simulink model "PSMG1"  (R2023b)
settings: Solver=ode23  StartTime=0.0  StopTime=1  FixedStep=0.0001  MaxStep=1e-4  RelTol=1e-3
undefined symbols (not defined in the file): J, Ke, Ld, Lq, p, Rs
settings Model: Creator=tudorn  LastModifiedBy=tudorn

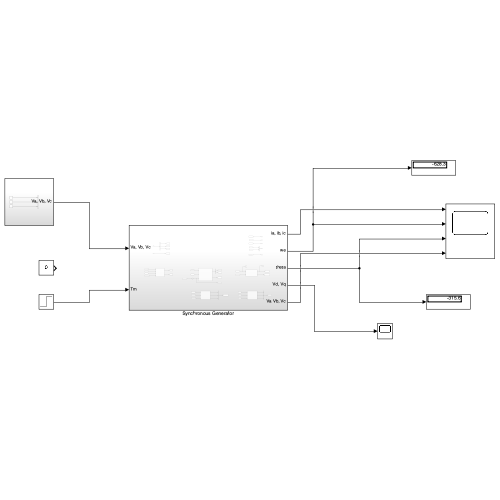
[thumbnail: Simulink's stored preview of the top-level diagram]
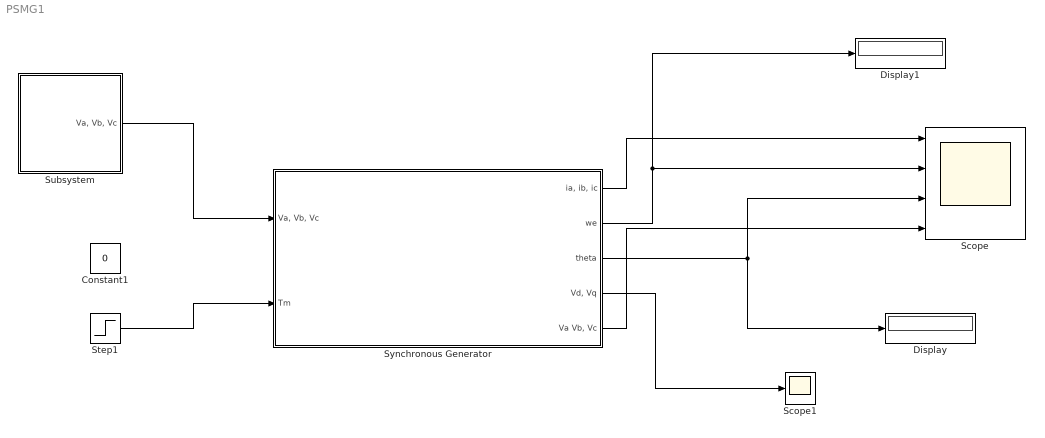
== system PSMG1 ==
  Constant1 : Constant  Value=0
  Display : Display
  Display1 : Display
  Scope : Scope  NumInputPorts=4
  Scope1 : Scope
  Step1 : Step  Time=0  After=3  SampleTime=0
  Subsystem : Subsystem
  Synchronous Generator : Subsystem
  wires:
  Subsystem/1("Va, Vb, Vc") -> Synchronous Generator/1("Va, Vb, Vc")
  Step1/1 -> Synchronous Generator/2(Tm)
  Synchronous Generator/1("ia, ib, ic") -> Scope/1
  Synchronous Generator/2(we) -> Display1/1, Scope/2
  Synchronous Generator/5("Va Vb, Vc") -> Scope/4
  Synchronous Generator/3(theta) -> Scope/3, Display/1
  Synchronous Generator/4("Vd, Vq") -> Scope1/1

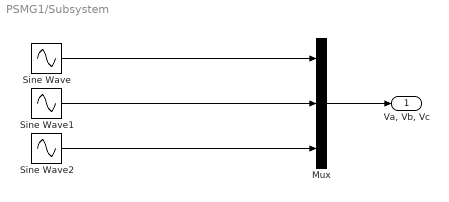
== system PSMG1/Subsystem ==
  Mux : Mux  Inputs=3
  Sine Wave : Sin  Amplitude=220  Frequency=2*pi*50  SampleTime=1e-5
  Sine Wave1 : Sin  Amplitude=220  Frequency=2*pi*50  Phase=2*pi/3  SampleTime=1e-5
  Sine Wave2 : Sin  Amplitude=220  Frequency=2*pi*50  Phase=-2*pi/3  SampleTime=1e-5
  "Va, Vb, Vc" : Outport
  wires:
  Mux/1 -> "Va, Vb, Vc"/1
  Sine Wave/1 -> Mux/1
  Sine Wave1/1 -> Mux/2
  Sine Wave2/1 -> Mux/3

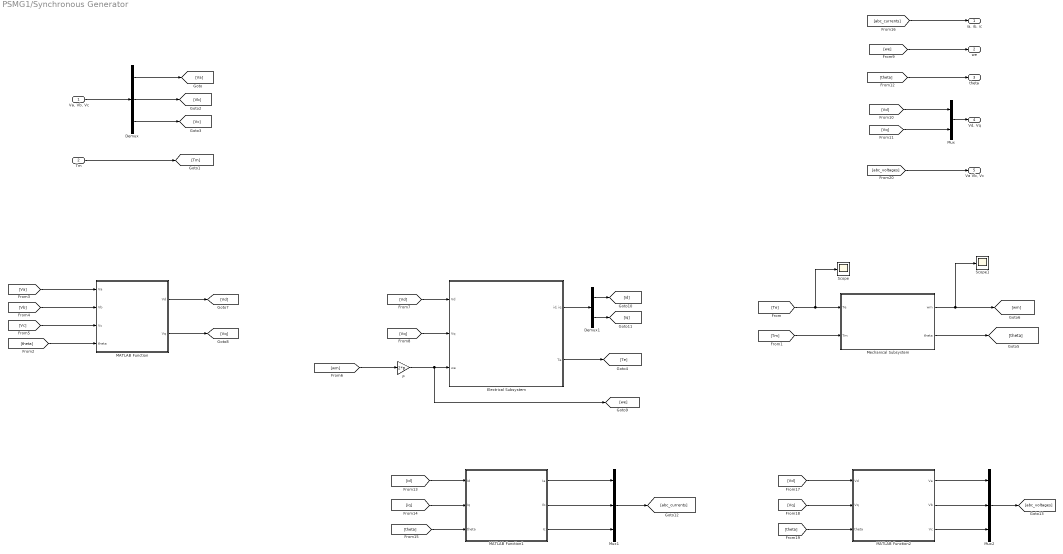
== system PSMG1/Synchronous Generator ==
  "Va, Vb, Vc" : Inport
  Tm : Inport  Port=2
  Demux : Demux  Outputs=3
  Demux1 : Demux  Outputs=2
  Electrical Subsystem : Subsystem
  MATLAB Function : MATLAB Function  TreatAsAtomicUnit=on
  MATLAB Function1 : MATLAB Function  TreatAsAtomicUnit=on
  MATLAB Function2 : MATLAB Function  TreatAsAtomicUnit=on
  Mechanical Subsystem : Subsystem
  Mux : Mux  Inputs=2
  Mux1 : Mux  Inputs=3
  Mux2 : Mux  Inputs=3
  P : Gain  Gain=2*p
  Scope : Scope
  Scope1 : Scope
  "ia, ib, ic" : Outport
  we : Outport  Port=2
  theta : Outport  Port=3
  "Vd, Vq" : Outport  Port=4
  "Va Vb, Vc" : Outport  Port=5
  wires:
  "Va, Vb, Vc"/1 -> Demux/1
  Tm/1 -> [Tm]
  Demux/1 -> [Va]
  Demux/2 -> [Vb]
  Demux/3 -> [Vc]
  Electrical Subsystem/2(Te) -> [Te]
  [Te] -> Scope/1, Mechanical Subsystem/1(Te)
  [Tm] -> Mechanical Subsystem/2(Tm)
  Mechanical Subsystem/2(theta) -> [theta]
  [theta] -> MATLAB Function/4(theta)
  [Vc] -> MATLAB Function/3(Vc)
  [Vb] -> MATLAB Function/2(Vb)
  [Va] -> MATLAB Function/1(Va)
  Mechanical Subsystem/1(wm) -> Scope1/1, [wm]
  [wm] -> P/1
  P/1 -> [we], Electrical Subsystem/3(we)
  [Vq] -> Electrical Subsystem/2(Vq)
  [Vd] -> Electrical Subsystem/1(Vd)
  MATLAB Function/1(Vd) -> [Vd]
  MATLAB Function/2(Vq) -> [Vq]
  [we] -> we/1
  Mux/1 -> "Vd, Vq"/1
  [Vd] -> Mux/1
  [Vq] -> Mux/2
  [theta] -> theta/1
  Electrical Subsystem/1("id, iq") -> Demux1/1
  Demux1/1 -> [id]
  Demux1/2 -> [iq]
  [iq] -> MATLAB Function1/2(Iq)
  [id] -> MATLAB Function1/1(Id)
  [theta] -> MATLAB Function1/3(theta)
  MATLAB Function1/1(Ia) -> Mux1/1
  MATLAB Function1/2(Ib) -> Mux1/2
  MATLAB Function1/3(Ic) -> Mux1/3
  Mux1/1 -> [abc_currents]
  [abc_currents] -> "ia, ib, ic"/1
  [Vd] -> MATLAB Function2/1(Vd)
  [Vq] -> MATLAB Function2/2(Vq)
  [theta] -> MATLAB Function2/3(theta)
  MATLAB Function2/1(Va) -> Mux2/1
  MATLAB Function2/2(Vb) -> Mux2/2
  MATLAB Function2/3(Vc) -> Mux2/3
  Mux2/1 -> [abc_voltages]
  [abc_voltages] -> "Va Vb, Vc"/1

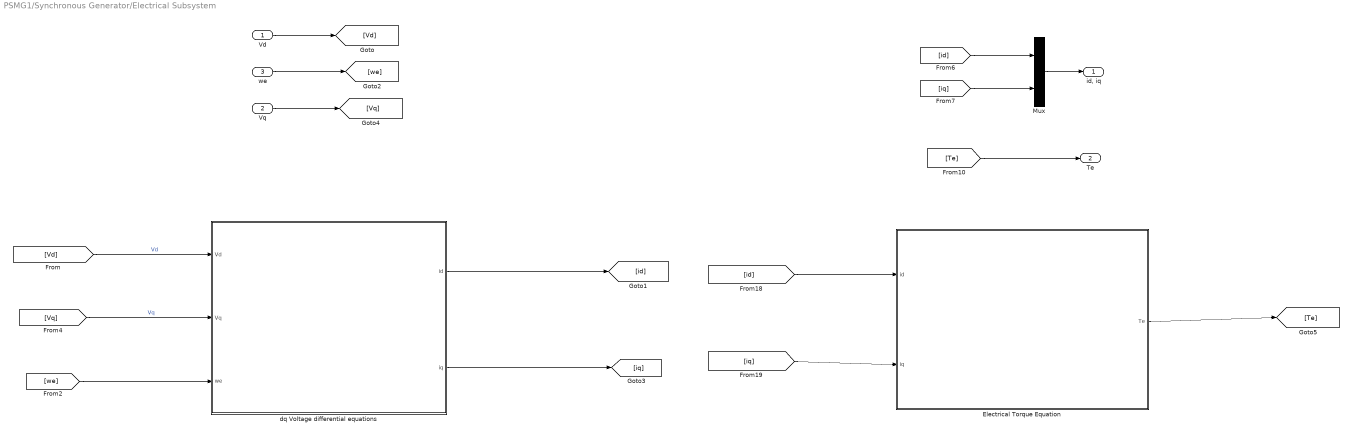
== system PSMG1/Synchronous Generator/Electrical Subsystem ==
  Vd : Inport
  Vq : Inport  Port=2
  we : Inport  Port=3
  Electrical Torque Equation : Subsystem
  Mux : Mux  Inputs=2
  dq Voltage differential equations : Subsystem
  "id, iq" : Outport
  Te : Outport  Port=2
  wires:
  Vd/1 -> [Vd]
  we/1 -> [we]
  Vq/1 -> [Vq]
  Mux/1 -> "id, iq"/1
  [id] -> Mux/1
  [iq] -> Mux/2
  [Te] -> Te/1
  [Vd] -> dq Voltage differential equations/1(Vd)  "Vd"
  [Vq] -> dq Voltage differential equations/2(Vq)  "Vq"
  dq Voltage differential equations/1(id) -> [id]
  dq Voltage differential equations/2(iq) -> [iq]
  [id] -> Electrical Torque Equation/1(id)
  [iq] -> Electrical Torque Equation/2(iq)
  Electrical Torque Equation/1(Te) -> [Te]
  [we] -> dq Voltage differential equations/3(we)

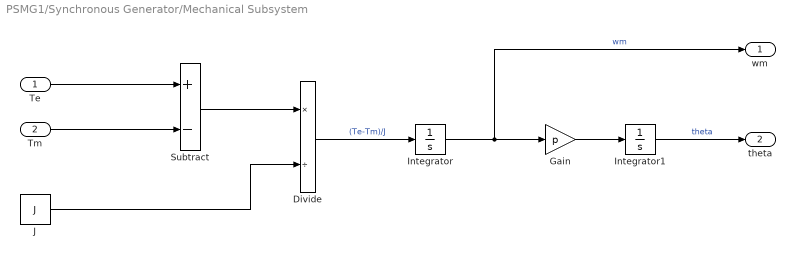
== system PSMG1/Synchronous Generator/Mechanical Subsystem ==
  Te : Inport
  Tm : Inport  Port=2
  Divide : Product  Inputs=*/
  Gain : Gain  Gain=p
  Integrator : Integrator
  Integrator1 : Integrator
  J : Constant  Value=J
  Subtract : Sum  Inputs=+-
  wm : Outport
  theta : Outport  Port=2
  wires:
  Tm/1 -> Subtract/2
  Te/1 -> Subtract/1
  Subtract/1 -> Divide/1
  J/1 -> Divide/2
  Divide/1 -> Integrator/1  "(Te-Tm)/J"
  Integrator/1 -> Gain/1, wm/1  "wm"
  Integrator1/1 -> theta/1  "theta"
  Gain/1 -> Integrator1/1

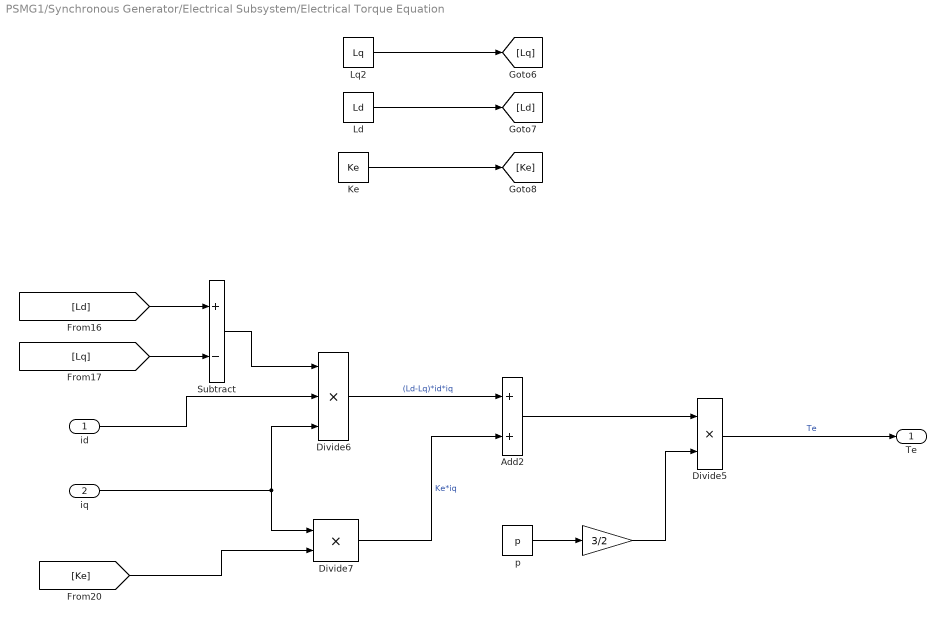
== system PSMG1/Synchronous Generator/Electrical Subsystem/Electrical Torque Equation ==
  id : Inport
  iq : Inport  Port=2
  " " : Gain  Gain=3/2
  Add2 : Sum
  Divide5 : Product  Inputs=**
  Divide6 : Product  Inputs=***
  Divide7 : Product  Inputs=**
  Ke : Constant  Value=Ke
  Ld : Constant  Value=Ld
  Lq2 : Constant  Value=Lq
  Subtract : Sum  Inputs=+-
  p : Constant  Value=p
  Te : Outport
  wires:
  id/1 -> Divide6/2
  [Ke] -> Divide7/2
  Divide5/1 -> Te/1  "Te"
  " "/1 -> Divide5/2
  iq/1 -> Divide7/1, Divide6/3
  [Ld] -> Subtract/1
  Subtract/1 -> Divide6/1
  p/1 -> " "/1
  Add2/1 -> Divide5/1
  Divide6/1 -> Add2/1  "(Ld-Lq)*id*iq"
  [Lq] -> Subtract/2
  Divide7/1 -> Add2/2  "Ke*iq"
  Ld/1 -> [Ld]
  Lq2/1 -> [Lq]
  Ke/1 -> [Ke]

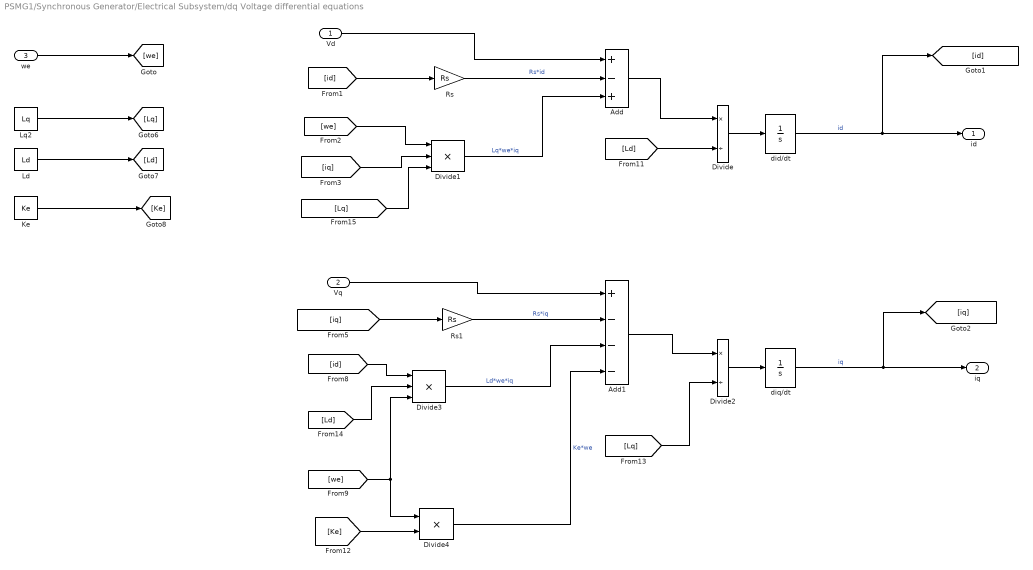
== system PSMG1/Synchronous Generator/Electrical Subsystem/dq Voltage differential equations ==
  Vd : Inport
  Vq : Inport  Port=2
  we : Inport  Port=3
  Add : Sum  Inputs=+-+
  Add1 : Sum  Inputs=+---
  Divide : Product  Inputs=*/
  Divide1 : Product  Inputs=***
  Divide2 : Product  Inputs=*/
  Divide3 : Product  Inputs=***
  Divide4 : Product  Inputs=**
  Ke : Constant  Value=Ke
  Ld : Constant  Value=Ld
  Lq2 : Constant  Value=Lq
  Rs : Gain  Gain=Rs
  Rs1 : Gain  Gain=Rs
  did/dt : Integrator
  diq/dt : Integrator
  id : Outport
  iq : Outport  Port=2
  wires:
  diq/dt/1 -> [iq], iq/1  "iq"
  Add/1 -> Divide/1
  did/dt/1 -> [id], id/1  "id"
  Rs1/1 -> Add1/2  "Rs*iq"
  [Lq] -> Divide2/2
  Vq/1 -> Add1/1
  [iq] -> Divide1/2
  [id] -> Divide3/1
  Divide1/1 -> Add/3  "Lq*we*iq"
  Add1/1 -> Divide2/1
  [iq] -> Rs1/1
  [Ld] -> Divide3/2
  Divide2/1 -> diq/dt/1
  [Lq] -> Divide1/3
  Rs/1 -> Add/2  "Rs*id"
  [we] -> Divide1/1
  Divide/1 -> did/dt/1
  [Ke] -> Divide4/2
  [we] -> Divide3/3, Divide4/1
  Divide4/1 -> Add1/4  "Ke*we"
  Divide3/1 -> Add1/3  "Ld*we*iq"
  [id] -> Rs/1
  Vd/1 -> Add/1
  [Ld] -> Divide/2
  Ld/1 -> [Ld]
  Lq2/1 -> [Lq]
  Ke/1 -> [Ke]
  we/1 -> [we]

== matlab function PSMG1/Synchronous Generator/MATLAB Function1 ==
  data: Id input; Ia output; Iq input; theta input; Ib output; Ic output
function [Ia, Ib, Ic] = Inverse_ClarkePark_Current(Id, Iq, theta)

    if isempty(theta)
        theta = 0;
    end

    Ia = Id * cos(theta) + Iq * sin(theta);
    Ib = Id * cos(theta - 2*pi/3) + Iq * sin(theta - 2*pi/3);
    Ic = Id * cos(theta + 2*pi/3) + Iq * sin(theta + 2*pi/3);

end

== matlab function PSMG1/Synchronous Generator/MATLAB Function ==
  data: Va input; Vd output; Vb input; Vc input; theta input; Vq output
function [Vd, Vq] = ClarkePark(Va, Vb, Vc, theta)

    if isempty(theta)
        theta = 0;
    end
    
    Vd = 2/3*(Va * cos(theta) + Vb * cos(theta-2*pi/3) + Vc * cos(theta+2*pi/3));
    Vq = 2/3*(Va * sin(theta) + Vb * sin(theta-2*pi/3) + Vc * sin(theta+2*pi/3));

end

== matlab function PSMG1/Synchronous Generator/MATLAB Function2 ==
  data: Vd input; Va output; Vq input; theta input; Vb output; Vc output
function [Va, Vb, Vc] = Inverse_ClarkePark_Voltage(Vd, Vq, theta)

    if isempty(theta)
        theta = 0;
    end

    Va = Vd * cos(theta) + Vq * sin(theta);
    Vb = Vd * cos(theta - 2*pi/3) + Vq * sin(theta - 2*pi/3);
    Vc = Vd * cos(theta + 2*pi/3) + Vq * sin(theta + 2*pi/3);

end
